simulink model "xiti4_13Step"  (Simulink 8.3)
settings: Solver=ode45  SolverMode=SingleTasking  StartTime=0.0  StopTime=10  FixedStep=0.25  RelTol=1e-3
values from neighbouring files (symbols this model uses):
  kd = kp*pi/(4*wr)    [xiti4_13Dm.m]    (also in xiti4_13Dm1.m)
  ki = kp*wr/pi    [xiti4_13Dm.m]    (also in xiti4_13Dm1.m)
  kp = 0.6*kr    [xiti4_13Dm.m]    (also in xiti4_13Dm1.m)
undefined symbols (not defined in the file or in its folder): DiscIntNeverNeededParam
settings Model: Creator=sony  LastModifiedBy=sony  ExtModeTrigMode=oneshot  ExtModeArmWhenConnect=off
settings DataIOCC: LimitDataPoints=off  SignalLoggingName=sigsOut
settings OptimizationCC: BooleanDataType=off
settings DebuggingCC: SaveWithParameterizedLinksMsg=none  SignalResolutionControl=TryResolveAllWithWarning  SolverPrmCheckMsg=none  MultiTaskDSMMsg=warning  MultiTaskCondExecSysMsg=none  StateNameClashWarn=none
settings HardwareCC: TargetUnknown=on
settings RTWCC: IncludeERTFirstTime=on

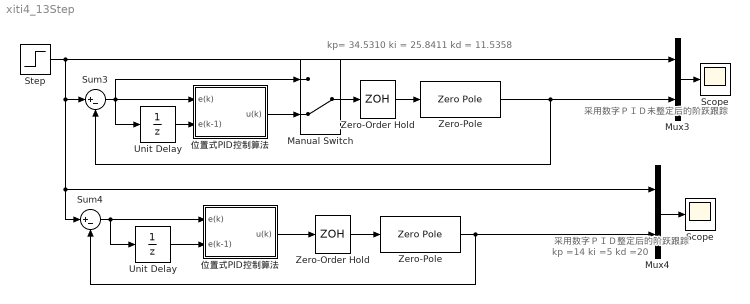
== system xiti4_13Step ==
  note: 采用数字ＰＩＤ未整定后的阶跃跟踪
  note: kp= 34.5310 ki = 25.8411 kd = 11.5358
  note: kp =14 ki =5 kd =20
  note: 采用数字ＰＩＤ整定后的阶跃跟踪
  "  Unit Delay " : UnitDelay  SampleTime=0.25
  "  Zero-Order Hold " : ZeroOrderHold  SampleTime=0.25
  "  Zero-Pole   " : ZeroPole  Zeros=[]  Poles=[-0.5 -0.2]  Gain=[0.1]
  " Scope " : Scope
      settings: YMin=-3.5  YMax=1  SaveName=ScopeData3  MaxDataPoints=500000
  " 位置式PID控制算法  " : Subsystem
  Manual Switch : ManualSwitch  CurrentSetting=0
  Mux3 : Mux  Inputs=2
  Mux4 : Mux  Inputs=2
  Scope : Scope
      settings: YMin=-3.5  YMax=1  SaveName=ScopeData2  MaxDataPoints=500000
  Step : Step  Time=0  SampleTime=0
  Sum3 : Sum  Inputs=|+-  SaturateOnIntegerOverflow=on
  Sum4 : Sum  Inputs=|+-  SaturateOnIntegerOverflow=on
  Unit Delay : UnitDelay  SampleTime=0.25
  Zero-Order Hold : ZeroOrderHold  SampleTime=0.25
  "Zero-Pole " : ZeroPole  Zeros=[]  Poles=[-0.5 -0.2]  Gain=[0.1]
  位置式PID控制算法 : Subsystem
  wires:
  Step/1 -> Sum3/1, Sum4/1, Mux4/1, Mux3/1
  Mux3/1 -> Scope/1
  "Zero-Pole "/1 -> Sum3/2, Mux3/2
  Unit Delay/1 -> 位置式PID控制算法/2(e(k-1))
  Sum3/1 -> Manual Switch/1, Unit Delay/1, 位置式PID控制算法/1(e(k))
  位置式PID控制算法/1(u(k)) -> Manual Switch/2
  Zero-Order Hold/1 -> "Zero-Pole "/1
  Manual Switch/1 -> Zero-Order Hold/1
  "  Zero-Pole   "/1 -> Mux4/2, Sum4/2
  "  Unit Delay "/1 -> " 位置式PID控制算法  "/2(e(k-1))
  Sum4/1 -> "  Unit Delay "/1, " 位置式PID控制算法  "/1(e(k))
  " 位置式PID控制算法  "/1(u(k)) -> "  Zero-Order Hold "/1
  "  Zero-Order Hold "/1 -> "  Zero-Pole   "/1
  Mux4/1 -> " Scope "/1

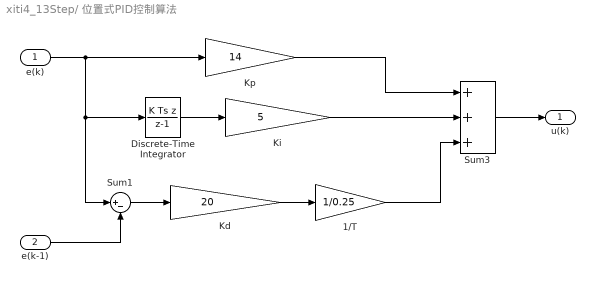
== system xiti4_13Step/ 位置式PID控制算法   ==
  e(k) : Inport
  e(k-1) : Inport  Port=2
  1/T : Gain  Gain=1/0.25  SaturateOnIntegerOverflow=on  OutDataTypeStr=Inherit: Same as input  ParamDataTypeStr=Inherit: Same as input
  Discrete-Time Integrator : DiscreteIntegrator  IntegratorMethod=Integration: Backward Euler  SampleTime=0.25  ICPrevOutput=DiscIntNeverNeededParam  ICPrevScaledInput=DiscIntNeverNeededParam
  Kd : Gain  Gain=20  SaturateOnIntegerOverflow=on  OutDataTypeStr=Inherit: Same as input  ParamDataTypeStr=Inherit: Same as input
  Ki : Gain  Gain=5  SaturateOnIntegerOverflow=on  OutDataTypeStr=Inherit: Same as input  ParamDataTypeStr=Inherit: Same as input
  Kp : Gain  Gain=14  SaturateOnIntegerOverflow=on  OutDataTypeStr=Inherit: Same as input  ParamDataTypeStr=Inherit: Same as input
  Sum1 : Sum  Inputs=|+-  SaturateOnIntegerOverflow=on
  Sum3 : Sum  Inputs=+++  SaturateOnIntegerOverflow=on
  u(k) : Outport
  wires:
  e(k-1)/1 -> Sum1/2
  1/T/1 -> Sum3/3
  Kd/1 -> 1/T/1
  Sum3/1 -> u(k)/1
  Ki/1 -> Sum3/2
  Kp/1 -> Sum3/1
  e(k)/1 -> Sum1/1, Discrete-Time Integrator/1, Kp/1
  Sum1/1 -> Kd/1
  Discrete-Time Integrator/1 -> Ki/1

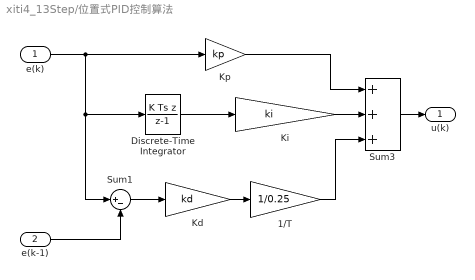
== system xiti4_13Step/位置式PID控制算法 ==
  e(k) : Inport
  e(k-1) : Inport  Port=2
  1/T : Gain  Gain=1/0.25  SaturateOnIntegerOverflow=on  OutDataTypeStr=Inherit: Same as input  ParamDataTypeStr=Inherit: Same as input
  Discrete-Time Integrator : DiscreteIntegrator  IntegratorMethod=Integration: Backward Euler  SampleTime=0.25  ICPrevOutput=DiscIntNeverNeededParam  ICPrevScaledInput=DiscIntNeverNeededParam
  Kd : Gain  Gain=kd  SaturateOnIntegerOverflow=on  OutDataTypeStr=Inherit: Same as input  ParamDataTypeStr=Inherit: Same as input
  Ki : Gain  Gain=ki  SaturateOnIntegerOverflow=on  OutDataTypeStr=Inherit: Same as input  ParamDataTypeStr=Inherit: Same as input
  Kp : Gain  Gain=kp  SaturateOnIntegerOverflow=on  OutDataTypeStr=Inherit: Same as input  ParamDataTypeStr=Inherit: Same as input
  Sum1 : Sum  Inputs=|+-  SaturateOnIntegerOverflow=on
  Sum3 : Sum  Inputs=+++  SaturateOnIntegerOverflow=on
  u(k) : Outport
  wires:
  e(k-1)/1 -> Sum1/2
  1/T/1 -> Sum3/3
  Kd/1 -> 1/T/1
  Sum3/1 -> u(k)/1
  Ki/1 -> Sum3/2
  Kp/1 -> Sum3/1
  e(k)/1 -> Sum1/1, Discrete-Time Integrator/1, Kp/1
  Sum1/1 -> Kd/1
  Discrete-Time Integrator/1 -> Ki/1
